simulink model "File_2_sim"  (Simulink 7.7)
settings: Solver=VariableStepDiscrete  StartTime=0.0  StopTime=5  RelTol=1e-3
libraries: powerlib_extras x2, dspsnks4 x1
settings Model: Creator=llokey  LastModifiedBy=kaman
settings OptimizationCC: InlineInvariantSignals=on  InitFltsAndDblsToZero=on
settings DebuggingCC: SaveWithParameterizedLinksMsg=none  SignalResolutionControl=TryResolveAllWithWarning  MultiTaskDSMMsg=warning  MultiTaskCondExecSysMsg=none  StrictBusMsg=None
settings RTWCC: IncludeERTFirstTime=on
settings GRTTargetCC: TargetFcnLib=ansi_tfl_tmw.mat

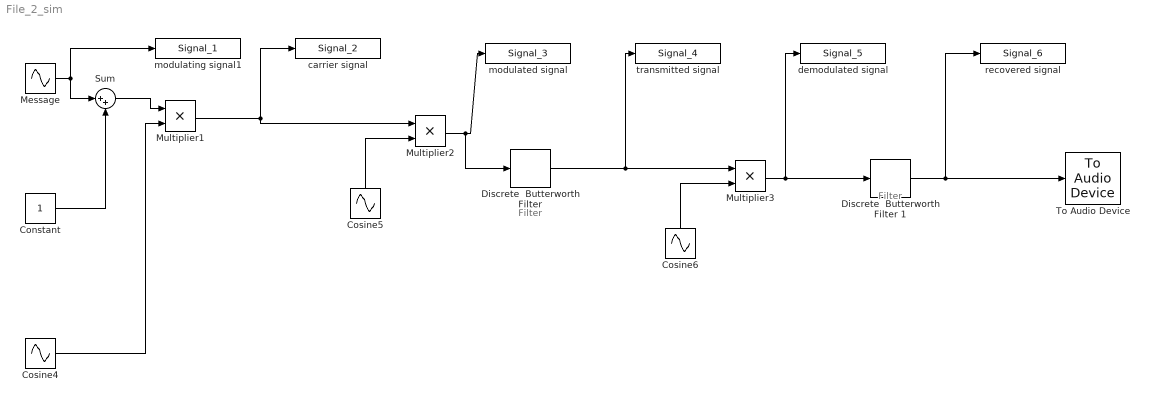
== system File_2_sim ==
  note: Filter
  note: Filter
  Constant : Constant
  Cosine4 : Sin  Frequency=2*pi*780  SampleTime=2e-5
  Cosine5 : Sin  Frequency=2*pi*1115  SampleTime=2e-5
  Cosine6 : Sin  Frequency=2*pi*335  SampleTime=2e-5
  "Discrete  Butterworth Filter " : powerlib_extras/Discrete  Control Blocks/Discrete  Butterworth Filter   SystemSampleTime=-1  FilterType=Bandpass  N=6  Fo=340  Bo=350  Ts=50e-6  Initialize=on  Vac_Init=[1.2 60 60]  Vdc_Init=-0.6  PlotResponse=off  param1=[1 500 0.1]
  Discrete  Butterworth Filter 1 : powerlib_extras/Discrete  Control Blocks/Discrete  Butterworth Filter   SystemSampleTime=-1  FilterType=Lowpass  N=6  Fo=10  Bo=10  Ts=50e-6  Initialize=on  Vac_Init=[1.2 60 60]  Vdc_Init=-0.6  PlotResponse=off  param1=[1 500 0.1]
  Message : Sin  Frequency=2*pi*1  SampleTime=2e-5
  Multiplier1 : Product  RndMeth=Zero
  Multiplier2 : Product  RndMeth=Zero
  Multiplier3 : Product  RndMeth=Zero
  Sum : Sum  Inputs=|++
  To Audio Device : dspsnks4/To Audio Device  deviceName=Default  inheritSampleRate=off  sampleRate=44100  deviceDatatype=Determine from input data type  autoBufferSize=on  bufferSize=4096  queueDuration=1.0
  carrier signal : ToWorkspace  VariableName=Signal_2  SampleTime=-1  SaveFormat=Structure With Time
  demodulated signal : ToWorkspace  VariableName=Signal_5  SampleTime=-1  SaveFormat=Structure With Time
  modulated signal : ToWorkspace  VariableName=Signal_3  SampleTime=-1  SaveFormat=Structure With Time
  modulating signal1 : ToWorkspace  VariableName=Signal_1  SampleTime=-1  SaveFormat=Structure With Time
  recovered signal : ToWorkspace  VariableName=Signal_6  SampleTime=-1  SaveFormat=Structure With Time
  transmitted signal : ToWorkspace  VariableName=Signal_4  SampleTime=-1  SaveFormat=Structure With Time
  wires:
  Cosine4/1 -> Multiplier1/2
  Multiplier1/1 -> carrier signal/1, Multiplier2/1
  Cosine5/1 -> Multiplier2/2
  Multiplier2/1 -> "Discrete  Butterworth Filter "/1, modulated signal/1
  Cosine6/1 -> Multiplier3/2
  "Discrete  Butterworth Filter "/1 -> Multiplier3/1, transmitted signal/1
  Message/1 -> Sum/1, modulating signal1/1
  Constant/1 -> Sum/2
  Sum/1 -> Multiplier1/1
  Multiplier3/1 -> Discrete  Butterworth Filter 1/1, demodulated signal/1
  Discrete  Butterworth Filter 1/1 -> To Audio Device/1, recovered signal/1
